simulink model "modulation"  (R2023a)
settings: Solver=VariableStepAuto  StartTime=0.0  StopTime=10.0  RelTol=1e-3
settings Model: Creator=prath  LastModifiedBy=prath

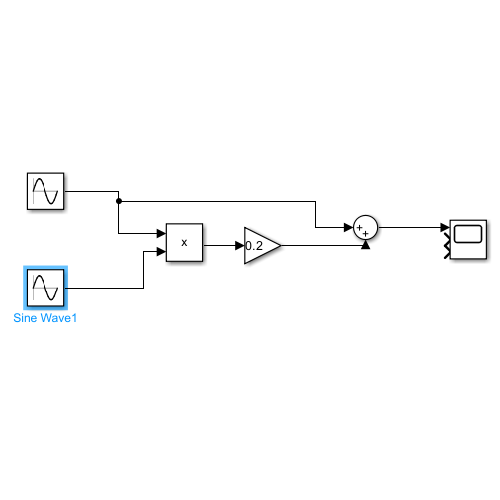
[thumbnail: Simulink's stored preview of the top-level diagram]
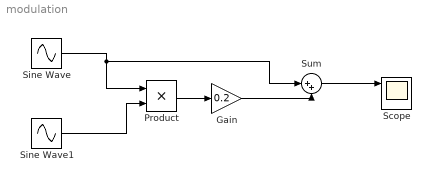
== system modulation ==
  Gain : Gain  Gain=0.2
  Product : Product
  Scope : Scope  NumInputPorts=3
  Sine Wave : Sin  Amplitude=5  Frequency=628.32  SampleTime=0
  Sine Wave1 : Sin  Frequency=6.28  SampleTime=0
  Sum : Sum  Inputs=|++
  wires:
  Sine Wave/1 -> Sum/1, Product/1
  Sine Wave1/1 -> Product/2
  Product/1 -> Gain/1
  Gain/1 -> Sum/2
  Sum/1 -> Scope/1
